simulink model "LKAS_AutoSave_20220310_1755"  (R2018b)
settings: Solver=FixedStepDiscrete  StartTime=0.0  StopTime=10.0  FixedStep=0.01  RelTol=1e-3
InitFcn:
  | tmpVer = ver('MATLAB');
  | tmpVer = str2num(tmpVer.Version);
  | % -------------------------------------------------------------------
  | %  MATLAB file generated by Simulink.saveVars on 21-Nov-2019 10:06:14
  | %  MATLAB version: 7.13.0.564 (R2011b)
  | % -------------------------------------------------------------------
  | 
  | 
  | SInt16 = Simulink.AliasType;
  | SInt16.Description = 'Num';
  | if (tmpVer > 7.11)
  | 	SInt16.DataScope = 'Auto';
  | end
  | SInt16.HeaderFile = 'Rte_Type.h';
  | SInt16.BaseType = 'int16';
  | 
  | SInt32 = Simulink.AliasType;
  | SInt32.Description = 'Num';
  | if (tmpVer > 7.11)
  | 	SInt32.DataScope = 'Auto';
  | end
  | SInt32.HeaderFile = 'Rte_Type.h';
  | SInt32.BaseType = 'int32';
  | 
  | SInt8 = Simulink.AliasType;
  | SInt8.Description = 'Num';
  | if (tmpVer > 7.11)
  | 	SInt8.DataScope = 'Auto';
  | end
  | SInt8.HeaderFile = 'Rte_Type.h';
  | SInt8.BaseType = 'int8';
  | 
  | T_A_m2_1024_1_u32 = Simulink.NumericType;
  | T_A_m2_1024_1_u32.Description = 'm2 (square meters  (m2))';
  | if (tmpVer > 7.11)
  | 	T_A_m2_1024_1_u32.DataScope = 'Auto';
  | end
  | T_A_m2_1024_1_u32.HeaderFile = 'Rte_Type.h';
  | T_A_m2_1024_1_u32.DataTypeMode = 'Fixed-point: slope and bias scaling';
  | T_A_m2_1024_1_u32.SignednessBool = false;
  | T_A_m2_1024_1_u32.WordLength = 32;
  | T_A_m2_1024_1_u32.FixedExponent = -10;
  | T_A_m2_1024_1_u32.SlopeAdjustmentFactor = 1;
  | T_A_m2_1024_1_u32.Bias = 0;
  | T_A_m2_1024_1_u32.DataTypeOverride = 'Inherit';
  | T_A_m2_1024_1_u32.IsAlias = true;
  | 
  | T_A_m2_65536_1_u16 = Simulink.NumericType;
  | T_A_m2_65536_1_u16.Description = 'm2 (square meters  (m2))';
  | if (tmpVer > 7.11)
  | 	T_A_m2_65536_1_u16.DataScope = 'Auto';
  | end
  | T_A_m2_65536_1_u16.HeaderFile = 'Rte_Type.h';
  | T_A_m2_65536_1_u16.DataTypeMode = 'Fixed-point: slope and bias scaling';
  | T_A_m2_65536_1_u16.SignednessBool = false;
  | T_A_m2_65536_1_u16.WordLength = 16;
  | T_A_m2_65536_1_u16.FixedExponent = -16;
  | T_A_m2_65536_1_u16.SlopeAdjustmentFactor = 1;
  | T_A_m2_65536_1_u16.Bias = 0;
  | T_A_m2_65536_1_u16.DataTypeOverride = 'Inherit';
  | ... (+4647 lines)
StopFcn:
  | clear  T_A_m2_1024_1_u32 T_A_m2_65536_1_u16 T_A_m2_Float32 T_A_mm2_10_1_u16 T_A_mm2_4_1_s16 T_A_mm2_Float32 T_Cnt_Num_10_1_u32 T_Cnt_Num_1_1_s16 T_Cnt_Num_1_1_s32 T_Cnt_Num_1_1_s8 T_Cnt_Num_1_1_u16 T_Cnt_Num_1_1_u32 T_Cnt_Num_1_1_u8 T_E_J_1_1_s32 T_E_J_Float32 T_E_kJ_128_1_s32 T_E_kJ_Float32 T_E_kwh_10_1_u16 T_E_kwh_Float32 T_Epl_kwhpkm_100_1_u16 T_Epl_kwhpkm_Float32 T_F_N_1_1_s16 T_F_N_Float32 T_I_A_1000_1_u16 T_I_A_1048576_1_s32 T_I_A_2048_1_s16 T_I_A_32_1_s16 T_I_A_Float32 T_I_mA_1_1_s16 T_I_mA_32768_128_s16 T_I_mA_Float32 T_J_kgpm2_128_1_u16 T_J_kgpm2_Float32 T_K_NA_1000_1_s16 T_K_NA_100_1_s16 T_K_NA_100_1_u16 T_K_NA_1024_1_s16 T_K_NA_1024_1_u16 T_K_NA_128_1_s16 T_K_NA_128_1_u16 T_K_NA_128_1_u8 T_K_NA_16777216_1_u32 T_K_NA_16_1_s16 T_K_NA_16_1_u16 T_K_NA_16_1_u8 T_K_NA_1_16_u16 T_K_NA_1_1_s16 T_K_NA_1_1_u16 T_K_NA_1_1_u8 T_K_NA_32768_1_s16 T_K_NA_32768_1_u16 T_K_NA_32_1_s8 T_K_NA_4096_1_u16 T_K_NA_4194304_1_s32 T_K_NA_4194304_1_u16 T_K_NA_65536_1_s32 T_K_NA_65536_1_u16 T_K_NA_8192_1_s16 T_K_NA_8_1_s16 T_K_NA_Float32 T_M_Nm_16_1_s16 T_M_Nm_1_1_s16 T_M_Nm_32768_1_s16 T_M_Nm_32_1_s16 T_M_Nm_4_1_s16 T_M_Nm_512_1_s16 T_M_Nm_Float32 T_P_W_1_4_s16 T_P_W_1_8_s16 T_P_W_Float32 T_P_kW_128_1_s16 T_P_kW_1_8_s16 T_P_kW_8_1_s32 T_P_kW_Float32 T_Pct_pct_1024_1_s32 T_Pct_pct_1024_1_u32 T_Pct_pct_10_1_s16 T_Pct_pct_10_1_u32 T_Pct_pct_128_100_s8 T_Pct_pct_1_1_s16 T_Pct_pct_1_4_u8 T_Pct_pct_255_100_u16 T_Pct_pct_255_100_u8 T_Pct_pct_256_1_s16 T_Pct_pct_256_1_u16 T_Pct_pct_65535_100_u16 T_Pct_pct_Float32 T_R_ohm_1024_1_s16 T_R_ohm_32_1_s16 T_R_ohm_Float32 T_TK_K_16_1_s16 T_TK_K_Float32 T_T_degC_10_400_1_u16 T_T_degC_16_1_s16 T_T_degC_1_40_1_u8 T_T_degC_2_80_1_u8 T_T_degC_Float32 T_U_V_1000_1_u16 T_U_V_10_1_u8 T_U_V_200_1_u8 T_U_V_32_1_s16 T_U_V_4096_1_s16 T_U_V_512_1_s16 T_U_V_65535_8_u16 T_U_V_8192_1_u16 T_U_V_Float32 T_U_mV_1_1_s16 T_U_mV_256_20_u16 T_U_mV_Float32 T_V_l_256_1_s16 T_V_l_4096_1_s16 T_V_l_64_1_s16 T_V_l_65535_100_u16 T_V_l_Float32 T_V_ml_128_1_s16 T_V_ml_1_1_s16 T_V_ml_32768_1_s16 T_V_ml_Float32 T_V_ul_32_1_u16 T_V_ul_Float32 T_Vpl_clpkm_512_1_u16 T_Vpl_clpkm_Float32 T_a_kphps_16_1_s16 T_a_kphps_Float32 T_a_mps2_128_1_s16 T_a_mps2_Float32 T_c_MJpkg_256_1_s16 T_c_MJpkg_Float32 T_c_kJpgpK_1024_1_s16 T_c_kJpgpK_Float32 T_c_kJpkgpK_128_1_u16 T_c_kJpkgpK_Float32 T_chrg_Ah_1_1_s16 T_chrg_Ah_1_1_u16 T_chrg_Ah_1_1_u8 T_chrg_Ah_256_1_u16 T_chrg_Ah_4194304_1_s32 T_chrg_Ah_512_1_u16 T_chrg_Ah_8_1_u16 T_chrg_Ah_Float32 T_cmp_NA_100_1_s16 T_cmp_NA_128_1_s16 T_cmp_NA_16_1_s16 T_cmp_NA_32768_1_u16 T_cmp_NA_Float32 T_d2n_rpmps2_4_1_s16 T_d2n_rpmps2_Float32 T_dPct_pctps_16_1_s16 T_dPct_pctps_256_1_s16 T_dPct_pctps_Float32 T_dT_degCps_128_1_s16 T_dT_degCps_Float32 T_dV_lph_1_1_s16 T_dV_lph_Float32 T_dV_lpm_128_1_s16 T_dV_lpm_32_1_s16 T_dV_lpm_Float32 T_dV_lps_1024_1_u16 T_dV_lps_4_1_u16 T_dV_lps_Float32 T_dV_mlps_1024_1_s16 T_dV_mlps_Float32 T_d_BitField16 T_dm_gps_128_1_s16 T_dm_gps_128_1_u16 T_dm_gps_256_1_u16 T_dm_gps_Float32 T_dm_mgps_1_1_s16 T_dm_mgps_Float32 T_dn_rpmps_1_1_s16 T_dn_rpmps_2_1_s16 T_dn_rpmps_Float32 T_dp_Paps_1_1_s16 T_dp_Paps_Float32 T_dp_kPaps_1_1_s16 T_dp_kPaps_8_1_s16 T_dp_kPaps_Float32 T_dphi_degps_128_1_s16 T_dphi_degps_8_1_s16 T_dphi_degps_Float32 T_dr_ps_256_1_s16 T_dr_ps_Float32 T_drho_mgplps_1_2_s16 T_drho_mgplps_Float32 T_e_NA_1_1_u8 T_f_Hz_1_1_u16 T_f_Hz_1_1_u32 T_f_Hz_64_1_u16 T_f_Hz_8_1_s16 T_f_Hz_Float32 T_g_BitField32 T_l_km_16_1_s16 T_l_km_1_1_u16 T_l_km_1_1_u32 T_l_km_Float32 T_l_m_1024_1_s16 T_l_m_16_1_s16 T_l_m_1_1_u32 T_l_m_Float32 T_l_mm_16_1_s16 T_l_mm_1_1_u16 T_l_mm_4096_1_s16 T_l_mm_4_1_u8 T_l_mm_64_1_s16 T_l_mm_Float32 T_m_g_1_1_s16 T_m_g_2048_1_s16 T_m_g_32_1_u16 T_m_g_Float32 T_m_kg_1024_1_s16 T_m_kg_1_1_s16 T_m_kg_1_1_u32 T_m_kg_Float32 T_m_mg_128_1_s16 T_m_mg_32_1_s16 T_m_mg_Float32 T_n_rpm_1_1_s16 T_n_rpm_1_25_u8 T_n_rpm_256_50_u16 T_n_rpm_2_25_u8 T_n_rpm_4_1_u16 T_n_rpm_Float32 T_p_MPa_64_1_s16 T_p_MPa_Float32 T_p_Pa_1_1_s16 T_p_Pa_Float32 T_p_kPa_1_10_u16 T_p_kPa_1_1_s16 T_p_kPa_1_1_u8 T_p_kPa_256_1_u16 T_p_kPa_32_1_u16 T_p_kPa_64_1_s16 T_p_kPa_Float32 T_phi_deg_100_1_s16 T_phi_deg_1024_1_s16 T_phi_deg_128_1_s16 T_phi_deg_1_1_u8 T_phi_deg_256_1_s16 T_phi_deg_2_1_s8 T_phi_deg_32_1_s16 T_phi_deg_512_6_s32 T_phi_deg_Float32 T_phi_rad_2048_1_s16 T_phi_rad_Float32 T_r_NA_1024_1_s16 T_r_NA_1024_1_u16 T_r_NA_16384_1_s16 T_r_NA_16_1_s16 T_r_NA_256_1_s8 T_r_NA_256_1_u16 T_r_NA_32768_1_u16 T_r_NA_32_1_u16 T_r_NA_4096_1_s16 T_r_NA_65535_2_u16 T_r_NA_8192_1_u16 T_r_NA_Float32 T_rho_gpl_8192_1_s16 T_rho_gpl_Float32 T_rho_kgpm3_16_1_s16 T_rho_kgpm3_Float32 T_rho_mgpl_1_1_s16 T_rho_mgpl_64_1_s16 T_rho_mgpl_Float32 T_t_hour_1_1_s16 T_t_hour_Float32 T_t_m_1_1_u16 T_t_m_Float32 T_t_ms_1_1_s16 T_t_ms_1_1_u16 T_t_ms_1_1_u32 T_t_ms_4096_1_s16 T_t_ms_64_1_s16 T_t_ms_Float32 T_t_s_1000_1_s16 T_t_s_100_1_s16 T_t_s_10_1_s16 T_t_s_10_1_u16 T_t_s_1_1_s16 T_t_s_1_1_u16 T_t_s_1_1_u32 T_t_s_Float32 T_t_us_10_1_u32 T_t_us_1_1_s16 T_t_us_1_1_u32 T_t_us_1_4_u16 T_t_us_Float32 T_v_kph_1_1_u8 T_v_kph_64_1_s16 T_v_kph_64_1_u16 T_v_kph_Float32 T_v_mps_256_1_s16 T_v_mps_Float32 T_w_radps_32_1_s16 T_w_radps_Float32 T_y_BitField8 T_y_BitFieldDiagProgress T_y_BitFieldDiagStatus T_y_NA_1_1_u8 SInt16 SInt32 SInt8 T_BOOLEAN UInt16 UInt32 UInt8 s16 s32 s8 u16 u32 u8
model workspace (MAT data in the model file):
  MCOS : class17 (value not decoded)
  MCOS : class17 (value not decoded)
  MCOS : class17 (value not decoded)
  MCOS : class17 (value not decoded)
  MCOS : class17 (value not decoded)
  MCOS : class17 (value not decoded)
  MCOS : class17 (value not decoded)
  MCOS : class17 (value not decoded)
  MCOS : class17 (value not decoded)
  MCOS : class17 (value not decoded)
  MCOS : class17 (value not decoded)
  MCOS : class17 (value not decoded)
  MCOS : class17 (value not decoded)
  MCOS : class17 (value not decoded)
  MCOS : class17 (value not decoded)
  MCOS : class17 (value not decoded)
  MCOS : class17 (value not decoded)
  MCOS : class17 (value not decoded)
  MCOS : class17 (value not decoded)
  MCOS : class17 (value not decoded)
  MCOS : class17 (value not decoded)
  MCOS : class17 (value not decoded)
  MCOS : class17 (value not decoded)
  MCOS : class17 (value not decoded)
  MCOS : class17 (value not decoded)
  MCOS : class17 (value not decoded)
  MCOS : class17 (value not decoded)
  MCOS : class17 (value not decoded)
  MCOS : class17 (value not decoded)
  MCOS : class17 (value not decoded)
  MCOS : class17 (value not decoded)
  MCOS : class17 (value not decoded)
  MCOS : class17 (value not decoded)
  MCOS : class17 (value not decoded)
  MCOS : class17 (value not decoded)
  MCOS : class17 (value not decoded)
  MCOS : class17 (value not decoded)
  MCOS : class17 (value not decoded)
  MCOS : class17 (value not decoded)
  MCOS : class17 (value not decoded)
  MCOS : class17 (value not decoded)
  MCOS : class17 (value not decoded)
  MCOS : class17 (value not decoded)
  MCOS : class17 (value not decoded)
  MCOS : class17 (value not decoded)
  MCOS : class17 (value not decoded)
  MCOS : class17 (value not decoded)
  MCOS : class17 (value not decoded)
  MCOS : class17 (value not decoded)
  MCOS : class17 (value not decoded)
  MCOS : class17 (value not decoded)
  MCOS : class17 (value not decoded)
  MCOS : class17 (value not decoded)
  MCOS : class17 (value not decoded)
  MCOS : class17 (value not decoded)
  MCOS : class17 (value not decoded)
  MCOS : class17 (value not decoded)
  MCOS : class17 (value not decoded)
  MCOS : class17 (value not decoded)
  MCOS : class17 (value not decoded)
  MCOS : class17 (value not decoded)
  MCOS : class17 (value not decoded)
  MCOS : class17 (value not decoded)
  MCOS : class17 (value not decoded)
  MCOS : class17 (value not decoded)
  MCOS : class17 (value not decoded)
  MCOS : class17 (value not decoded)
  MCOS : class17 (value not decoded)
  MCOS : class17 (value not decoded)
  MCOS : class17 (value not decoded)
  MCOS : class17 (value not decoded)
  MCOS : class17 (value not decoded)
  MCOS : class17 (value not decoded)
  MCOS : class17 (value not decoded)
  MCOS : class17 (value not decoded)
  MCOS : class17 (value not decoded)
  MCOS : class17 (value not decoded)
  MCOS : class17 (value not decoded)
  MCOS : class17 (value not decoded)
  MCOS : class17 (value not decoded)
  MCOS : class17 (value not decoded)
  MCOS : class17 (value not decoded)
  MCOS : class17 (value not decoded)
  MCOS : class17 (value not decoded)
  MCOS : class17 (value not decoded)
  MCOS : class17 (value not decoded)
  MCOS : class17 (value not decoded)
  MCOS : class17 (value not decoded)
  MCOS : class17 (value not decoded)
  MCOS : class17 (value not decoded)
  MCOS : class17 (value not decoded)
  MCOS : class17 (value not decoded)
  MCOS : class17 (value not decoded)
  MCOS : class17 (value not decoded)
  MCOS : class17 (value not decoded)
  MCOS : class17 (value not decoded)
  MCOS : class17 (value not decoded)
  MCOS : class17 (value not decoded)
  MCOS : class17 (value not decoded)
  MCOS : class17 (value not decoded)
  MCOS : class17 (value not decoded)
  MCOS : class17 (value not decoded)
undefined symbols (not defined in the file): LKA_CarWidth, LKA_SampleTime, LKA_StrRatio_C, LKA_Veh2CamL_C, LKA_Veh2CamW_C, LKA_WhlBaseL_C, LL_CompHdAg_C, LL_CompSWA_C, LL_CrvtPrvwT_C, LL_DesDvt_C, LL_DvtComp_C, LL_DvtPrvwT_C, LL_DvtSpdDet_vDvtSpdMin_C, LL_HandsOff_ExitTime, LL_HandsOff_TextTime, LL_HandsOff_WarnTime, LL_HdAgExT_C, LL_HdAgPrvwT_C, LL_LAccMax_C, LL_LAccRMax_C, LL_LDW_EarliestWarnLine_C, LL_LDW_LatestWarnLine_C, LL_LDWS_SUPPRESS_HEADING, LL_LFClb_TFC_FfCtlRatio_C, LL_LFClb_TFC_KdBalance_C, LL_LFClb_TFC_KdMaxSWA_C, LL_LFClb_TFC_KdV1_C, LL_LFClb_TFC_KdV2_C, LL_LFClb_TFC_KdVehSpdLwr_C, LL_LFClb_TFC_KdVehSpdUpr_C, LL_LFClb_TFC_Ki_C, LL_LFClb_TFC_KiMaxSWA_C, LL_LFClb_TFC_Kp_C, LL_LFClb_TFC_KpKlat_C, LL_LFClb_TFC_KpV1_C, LL_LFClb_TFC_KpV2_C, LL_LFClb_TFC_KpVehSpdLwr_C, LL_LFClb_TFC_KpVehSpdUpr_C, LL_LFClb_TFC_PrvwT_C, LL_LKA_EarliestWarnLine_C, LL_LKA_LatestWarnLine_C, LL_LKAExPrcs_ExitC0Dvt, LL_LKAExPrcs_ExitC0Swt, LL_LKAExPrcs_tiExitTime1, LL_LKAExPrcs_tiExitTime2, LL_LKAExPrcs_tiExitTime3, LL_LKAS_OUT_OF_CONTROL_LAT_VEL, LL_LKAS_OUT_OF_CONTROL_TTLC, LL_LKASWASyn_M0, LL_LKASWASyn_M1, LL_LKASWASyn_M2, LL_LKASWASyn_M3K, LL_LKASWASyn_SWAaddMax, LL_LKASWASyn_T2, LL_LKASWASyn_tiTrqSwaRtTime, LL_LKASWASyn_tiTrqSwaTime, LL_LKASWASyn_TrqMax, LL_LKASWASyn_TrqSwaAddSwt, LL_LKASWASyn_TrqSwaRateDiff, LL_LSpdCompT_C ... (+43)
libraries: simulink x138, canmsglib x8, dspstat3 x3, simulink_extras x1
(part 6 of 20)

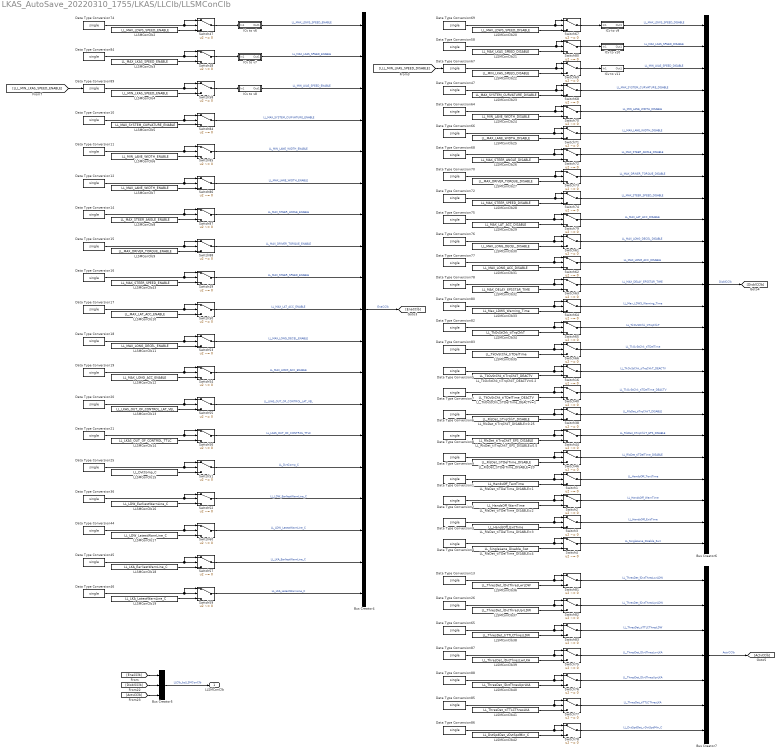
== system LKAS_AutoSave_20220310_1755/LKAS/LLClb/LLSMConClb ==
  Bus Creator4 : BusCreator  Inputs=19
  Bus Creator5 : BusCreator  Inputs=3
  Bus Creator6 : BusCreator  Inputs=25
  Bus Creator7 : BusCreator  Inputs=7
  Data Type Conversion{1..21,25..26,36,44..47,58,64..70,72,74..78,80,82..89} (51 alike) : DataTypeConversion  OutDataTypeStr=single
  ICv to v10 : Subsystem
  ICv to v11 : Subsystem
  ICv to v6 : Subsystem  Description=|
      | 仪表车速转换
      | 仪表车速 = 实际车速 * 1.02 + 2.5
      settings: AttributesFormatString=%<Description>
  ICv to v7 : Subsystem
  ICv to v8 : Subsystem
  ICv to v9 : Subsystem
  LLSMConClb10 : Constant  Description=侧向加速度使能上限  Value=LL_MAX_LAT_ACC_ENABLE  OutDataTypeStr=single
      settings: AttributesFormatString=|
      | %<Value>  = 3
      | %<Description>
  LLSMConClb11 : Constant  Description=纵向减速度使能上限  Value=LL_MAX_LONG_DECEL_ENABLE  OutDataTypeStr=single
      settings: AttributesFormatString=|
      | %<Value>  = 2
      | %<Description>
  LLSMConClb12 : Constant  Description=纵向加速度使能上限  Value=LL_MAX_LONG_ACC_ENABLE  OutDataTypeStr=single
      settings: AttributesFormatString=|
      | %<Value>  = 3
      | %<Description>
  LLSMConClb13 : Constant  Description=LKA功能的侧向偏出速度阈值  Value=LL_LKAS_OUT_OF_CONTROL_LAT_VEL  OutDataTypeStr=single
      settings: AttributesFormatString=|
      | %<Value>  = 1.5
      | %<Description>
  LLSMConClb14 : Constant  Description=LKA功能的超过最迟干预线持续时间阈值  Value=LL_LKAS_OUT_OF_CONTROL_TTLC  OutDataTypeStr=single
      settings: AttributesFormatString=|
      | %<Value>  = 0.3
      | %<Description>
  LLSMConClb15 : Constant  Description=偏移量补偿  Value=LL_DvtComp_C  OutDataTypeStr=single
      settings: AttributesFormatString=|
      | %<Value>  = 0
      | %<Description>
  LLSMConClb16 : Constant  Description=LDW功能的最早预警线  Value=LL_LDW_EarliestWarnLine_C  OutDataTypeStr=single
      settings: AttributesFormatString=|
      | %<Value>  = 0.3
      | %<Description>
  LLSMConClb17 : Constant  Description=LDW功能的最迟预警线  Value=LL_LDW_LatestWarnLine_C  OutDataTypeStr=single
      settings: AttributesFormatString=|
      | %<Value>  = -0.4
      | %<Description>
  LLSMConClb18 : Constant  Description=LKA功能的最早预警线  Value=LL_LKA_EarliestWarnLine_C  OutDataTypeStr=single
      settings: AttributesFormatString=|
      | %<Value>  = 0.3
      | %<Description>
  LLSMConClb19 : Constant  Description=LKA功能的最迟预警线  Value=LL_LKA_LatestWarnLine_C  OutDataTypeStr=single
      settings: AttributesFormatString=|
      | %<Value>  = -0.5
      | %<Description>
  LLSMConClb2 : Constant  Description=LDW功能的车速使能上限  Value=LL_MAX_LDWS_SPEED_ENABLE  OutDataTypeStr=single
      settings: AttributesFormatString=|
      | %<Value>  = 140
      | %<Description>
  LLSMConClb20 : Constant  Description=LDW功能的车速失效上限  Value=LL_MAX_LDWS_SPEED_DISABLE  OutDataTypeStr=single
      settings: AttributesFormatString=|
      | %<Value>  = 150
      | %<Description>
  LLSMConClb21 : Constant  Description=LKA功能的车速失效上限  Value=LL_MAX_LKAS_SPEED_DISABLE  OutDataTypeStr=single
      settings: AttributesFormatString=|
      | %<Value>  = 150
      | %<Description>
  LLSMConClb22 : Constant  Description=LKA功能的车速失效下限  Value=LL_MIN_LKAS_SPEED_DISABLE  OutDataTypeStr=single
      settings: AttributesFormatString=|
      | %<Value>  = 55
      | %<Description>
  LLSMConClb23 : Constant  Description=曲率失效上限  Value=LL_MAX_SYSTEM_CURVATURE_DISABLE  OutDataTypeStr=single
      settings: AttributesFormatString=|
      | %<Value>  = 0.0055
      | %<Description>
  LLSMConClb24 : Constant  Description=车道线宽度失效下限  Value=LL_MIN_LANE_WIDTH_DISABLE  OutDataTypeStr=single
      settings: AttributesFormatString=|
      | %<Value>  = 2.4
      | %<Description>
  LLSMConClb25 : Constant  Description=车道线宽度失效上限  Value=LL_MAX_LANE_WIDTH_DISABLE  OutDataTypeStr=single
      settings: AttributesFormatString=|
      | %<Value>  = 5.5
      | %<Description>
  LLSMConClb26 : Constant  Description=方向盘转角退出上限  Value=LL_MAX_STEER_ANGLE_DISABLE  OutDataTypeStr=single
      settings: AttributesFormatString=|
      | %<Value>  = 70
      | %<Description>
  LLSMConClb27 : Constant  Description=驾驶员转矩失效上限  Value=LL_MAX_DRIVER_TORQUE_DISABLE  OutDataTypeStr=single
      settings: AttributesFormatString=|
      | %<Value>  = 2.25
      | %<Description>
  LLSMConClb28 : Constant  Description=方向盘转速失效上限  Value=LL_MAX_STEER_SPEED_DISABLE  OutDataTypeStr=single
      settings: AttributesFormatString=|
      | %<Value>  = 5000
      | %<Description>
  LLSMConClb29 : Constant  Description=侧向加速度失效上限  Value=LL_MAX_LAT_ACC_DISABLE  OutDataTypeStr=single
      settings: AttributesFormatString=|
      | %<Value>  = 3.5
      | %<Description>
  LLSMConClb3 : Constant  Description=LKA功能的车速使能上限  Value=LL_MAX_LKAS_SPEED_ENABLE  OutDataTypeStr=single
      settings: AttributesFormatString=|
      | %<Value>  = 140
      | %<Description>
  LLSMConClb30 : Constant  Description=纵向减速度失效上限  Value=LL_MAX_LONG_DECEL_DISABLE  OutDataTypeStr=single
      settings: AttributesFormatString=|
      | %<Value>  = 2.5
      | %<Description>
  LLSMConClb31 : Constant  Description=纵向加速度失效上限  Value=LL_MAX_LONG_ACC_DISABLE  OutDataTypeStr=single
      settings: AttributesFormatString=|
      | %<Value>  = 3.5
      | %<Description>
  LLSMConClb32 : Constant  Description=LKA功能的EPS延迟进入等待的时间上限  Value=LL_MAX_DELAY_EPSSTAR_TIME  OutDataTypeStr=single
      settings: AttributesFormatString=|
      | %<Value>  = 0.5
      | %<Description>
  LLSMConClb33 : Constant  Description=LDW功能的连续报警时间上限  Value=LL_Max_LDWS_Warning_Time  OutDataTypeStr=single
      settings: AttributesFormatString=|
      | %<Value>  = 5
      | %<Description>
  LLSMConClb34 : Constant  Description=驾驶员接管时间阈值  Value=LL_TkOvStChk_tiTrqChkT  OutDataTypeStr=single
      settings: AttributesFormatString=|
      | %<Value>  = 0.1
      | %<Description>
  LLSMConClb35 : Constant  Description=距离上次驾驶员接管时间间隔  Value=LL_TkOvStChk_tiTDelTime  OutDataTypeStr=single
      settings: AttributesFormatString=|
      | %<Value>  = 2
      | %<Description>
  LLSMConClb36 : Constant  Description=LDW功能的偏移量激活下限  Value=LL_ThresDet_lDvtThresLwrLDW  OutDataTypeStr=single
      settings: AttributesFormatString=|
      | %<Value>  = 0.15
      | %<Description>
  LLSMConClb37 : Constant  Description=LDW功能的偏移量激活上限  Value=LL_ThresDet_lDvtThresUprLDW  OutDataTypeStr=single
      settings: AttributesFormatString=|
      | %<Value>  = 0.3
      | %<Description>
  LLSMConClb38 : Constant  Description=LDW功能的跨道时间激活阈值  Value=LL_ThresDet_tiTTLCThresLDW  OutDataTypeStr=single
      settings: AttributesFormatString=|
      | %<Value>  = 0.75
      | %<Description>
  LLSMConClb39 : Constant  Description=LKA功能的偏移量激活下限  Value=LL_ThresDet_lDvtThresLwrLKA  OutDataTypeStr=single
      settings: AttributesFormatString=|
      | %<Value>  = 0.3
      | %<Description>
  LLSMConClb4 : Constant  Description=LKA功能的车速使能下限  Value=LL_MIN_LKAS_SPEED_ENABLE  OutDataTypeStr=single
      settings: AttributesFormatString=|
      | %<Value>  = 60
      | %<Description>
  LLSMConClb40 : Constant  Description=LKA功能的偏移量激活上限  Value=LL_ThresDet_lDvtThresUprLKA  OutDataTypeStr=single
      settings: AttributesFormatString=|
      | %<Value>  = 0.6
      | %<Description>
  LLSMConClb41 : Constant  Description=LKA功能的跨道时间激活阈值  Value=LL_ThresDet_tiTTLCThresLKA  OutDataTypeStr=single
      settings: AttributesFormatString=|
      | %<Value>  = 1.5
      | %<Description>
  LLSMConClb42 : Constant  Description=偏出侧向速度最小值  Value=LL_DvtSpdDet_vDvtSpdMin_C  OutDataTypeStr=single
      settings: AttributesFormatString=|
      | %<Value>  = 0
      | %<Description>
  LLSMConClb43 : Constant  Description=方向盘转速使能上限  Value=LL_MAX_STEER_SPEED_ENABLE  OutDataTypeStr=single
      settings: AttributesFormatString=|
      | %<Value>  = 5000
      | %<Description>
  LLSMConClb5 : Constant  Description=曲率使能上限  Value=LL_MAX_SYSTEM_CURVATURE_ENABLE  OutDataTypeStr=single
      settings: AttributesFormatString=|
      | %<Value>  = 0.0045
      | %<Description>
  LLSMConClb6 : Constant  Description=车道线宽度使能下限  Value=LL_MIN_LANE_WIDTH_ENABLE  OutDataTypeStr=single
      settings: AttributesFormatString=|
      | %<Value>  = 2.5
      | %<Description>
  LLSMConClb7 : Constant  Description=车道线宽度使能上限  Value=LL_MAX_LANE_WIDTH_ENABLE  OutDataTypeStr=single
      settings: AttributesFormatString=|
      | %<Value>  = 5.4
      | %<Description>
  LLSMConClb8 : Constant  Description=方向盘转角使能上限  Value=LL_MAX_STEER_ANGLE_ENABLE  OutDataTypeStr=single
      settings: AttributesFormatString=|
      | %<Value>  = 60
      | %<Description>
  LLSMConClb9 : Constant  Description=驾驶员扭矩使能上限  Value=LL_MAX_DRIVER_TORQUE_ENABLE  OutDataTypeStr=single
      settings: AttributesFormatString=|
      | %<Value>  = 3
      | %<Description>
  LL_RlsDet_tiTDelTime_DISABLE=1 : Constant  Description=驾驶员脱手开始到功能发出动画提醒的时间  Value=LL_HandsOff_TextTime  OutDataTypeStr=single
      settings: AttributesFormatString=|
      | %<Value>  = 10
      | %<Description>
  LL_RlsDet_tiTDelTime_DISABLE=2 : Constant  Description=驾驶员脱手开始到发出声音报警的时间  Value=LL_HandsOff_WarnTime  OutDataTypeStr=single
      settings: AttributesFormatString=|
      | %<Value>  = 15
      | %<Description>
  LL_RlsDet_tiTDelTime_DISABLE=20 : Constant  Description=反使能距离上次驾驶员脱手时间间隔  Value=LL_RlsDet_tiTDelTime_DISABLE  OutDataTypeStr=single
      settings: AttributesFormatString=|
      | %<Value>  = 20
      | %<Description>
  LL_RlsDet_tiTDelTime_DISABLE=3 : Constant  Description=驾驶员脱手开始到功能退出的时间  Value=LL_HandsOff_ExitTime  OutDataTypeStr=single
      settings: AttributesFormatString=|
      | %<Value>  = 20
      | %<Description>
  LL_RlsDet_tiTDelTime_DISABLE=4 : Constant  Description=驾驶员脱手开始到功能退出的时间  Value=LL_SingleLane_Disable_Swt  OutDataTypeStr=boolean
      settings: AttributesFormatString=|
      | %<Value>  = 0
      | %<Description>
  LL_RlsDet_tiTrqChkT_DISABLE=0.25 : Constant  Description=反使能驾驶员脱手时间阈值  Value=LL_RlsDet_tiTrqChkT_DISABLE  OutDataTypeStr=single
      settings: AttributesFormatString=|
      | %<Value>  = 0.25
      | %<Description>
  LL_RlsDet_tiTrqChkT_EPS_DISABLE=0.5 : Constant  Description=反使能驾驶员脱手时间阈值（EPS激活）  Value=LL_RlsDet_tiTrqChkT_EPS_DISABLE  OutDataTypeStr=single
      settings: AttributesFormatString=|
      | %<Value>  = 0.5
      | %<Description>
  LL_TkOvStChk_tiTDelTime_DEACTV=1 : Constant  Description=取消激活距离上次驾驶员接管时间间隔  Value=LL_TkOvStChk_tiTDelTime_DEACTV  OutDataTypeStr=single
      settings: AttributesFormatString=|
      | %<Value>  = 1
      | %<Description>
  LL_TkOvStChk_tiTrqChkT_DEACTV=0.2 : Constant  Description=取消激活驾驶员接管时间阈值  Value=LL_TkOvStChk_tiTrqChkT_DEACTV  OutDataTypeStr=single
      settings: AttributesFormatString=|
      | %<Value>  = 0.2
      | %<Description>
  Switch{1..3,16,38,40,44,46..88} (50 alike) : Switch  Criteria=u2 ~= 0  OutDataTypeStr=single
  Switch4 : Switch  Criteria=u2 ~= 0  OutDataTypeStr=boolean
  LLSMConClb : Outport
  wires:
  Bus Creator5/1 -> LLSMConClb/1  "LLClb_bsLLSMConClb"
  [ActvCClb] -> Bus Creator5/3
  [DisblCClb] -> Bus Creator5/2
  [EnaCClb] -> Bus Creator5/1
  ICv to v6/1(Out1) -> Bus Creator4/1  "LL_MAX_LDWS_SPEED_ENABLE"
  LLSMConClb3/1 -> Switch48/3
  LLSMConClb10/1 -> Switch50/3
  LLSMConClb41/1 -> Switch77/3
  Data Type Conversion66/1 -> Switch71/1, Switch71/2
  LLSMConClb39/1 -> Switch75/3
  LLSMConClb11/1 -> Switch53/3
  LLSMConClb12/1 -> Switch54/3
  Switch55/1 -> Bus Creator4/13  "LL_LKAS_OUT_OF_CONTROL_LAT_VEL"
  Switch82/1 -> Bus Creator7/2  "LL_ThresDet_lDvtThresUprLDW"
  Data Type Conversion46/1 -> Switch59/1, Switch59/2
  Bus Creator7/1 -> [ActvCClb]  "ActvCClb"
  [LLL_MIN_LKAS_SPEED_DISABLE] -> Data Type Conversion67/1
  Data Type Conversion65/1 -> Switch83/2, Switch83/1
  ICv to v9/1(Out1) -> Bus Creator6/1  "LL_MAX_LDWS_SPEED_DISABLE"
  Switch69/1 -> ICv to v11/1(In1)
  LLSMConClb38/1 -> Switch83/3
  Data Type Conversion17/1 -> Switch50/1, Switch50/2
  Data Type Conversion78/1 -> Switch63/1, Switch63/2
  Data Type Conversion14/1 -> Switch87/1, Switch87/2
  ICv to v7/1(Out1) -> Bus Creator4/2  "LL_MAX_LKAS_SPEED_ENABLE"
  LLSMConClb35/1 -> Switch66/3
  Data Type Conversion64/1 -> Switch70/1, Switch70/2
  LLSMConClb14/1 -> Switch56/3
  Data Type Conversion69/1 -> Switch67/1, Switch67/2
  LLSMConClb5/1 -> Switch84/3
  LLSMConClb37/1 -> Switch82/3
  Data Type Conversion70/1 -> Switch73/1, Switch73/2
  Switch85/1 -> Bus Creator4/5  "LL_MIN_LANE_WIDTH_ENABLE"
  LLSMConClb23/1 -> Switch68/3
  Switch59/1 -> Bus Creator4/19  "LL_LKA_LatestWarnLine_C"
  LLSMConClb25/1 -> Switch71/3
  LLSMConClb43/1 -> Switch49/3
  Switch49/1 -> Bus Creator4/9  "LL_MAX_STEER_SPEED_ENABLE"
  LLSMConClb40/1 -> Switch76/3
  Switch50/1 -> Bus Creator4/10  "LL_MAX_LAT_ACC_ENABLE"
  Data Type Conversion68/1 -> Switch72/1, Switch72/2
  LLSMConClb33/1 -> Switch64/3
  Switch81/1 -> Bus Creator7/1  "LL_ThresDet_lDvtThresLwrLDW"
  Data Type Conversion18/1 -> Switch53/1, Switch53/2
  Switch84/1 -> Bus Creator4/4  "LL_MAX_SYSTEM_CURVATURE_ENABLE"
  Data Type Conversion76/1 -> Switch61/2, Switch61/1
  Switch53/1 -> Bus Creator4/11  "LL_MAX_LONG_DECEL_ENABLE"
  Data Type Conversion11/1 -> Switch85/1, Switch85/2
  LLSMConClb27/1 -> Switch73/3
  Data Type Conversion84/1 -> Switch48/1, Switch48/2
  Switch70/1 -> Bus Creator6/5  "LL_MIN_LANE_WIDTH_DISABLE"
  LLSMConClb34/1 -> Switch65/3
  Data Type Conversion16/1 -> Switch49/1, Switch49/2
  Switch64/1 -> Bus Creator6/14  "LL_Max_LDWS_Warning_Time"
  Data Type Conversion88/1 -> Switch76/1, Switch76/2
  Data Type Conversion13/1 -> Switch81/1, Switch81/2
  Switch52/1 -> Bus Creator4/16  "LL_LDW_EarliestWarnLine_C"
  Switch79/1 -> Bus Creator6/10  "LL_MAX_LAT_ACC_DISABLE"
  Data Type Conversion72/1 -> Switch74/1, Switch74/2
  LLSMConClb18/1 -> Switch57/3
  Data Type Conversion82/1 -> Switch65/1, Switch65/2
  Data Type Conversion58/1 -> Switch80/1, Switch80/2
  Data Type Conversion19/1 -> Switch54/1, Switch54/2
  Switch51/1 -> Bus Creator4/15  "LL_DvtComp_C"
  Switch76/1 -> Bus Creator7/5  "LL_ThresDet_lDvtThresUprLKA"
  LLSMConClb7/1 -> Switch86/3
  Switch48/1 -> ICv to v7/1(In1)
  Data Type Conversion36/1 -> Switch52/1, Switch52/2
  Switch63/1 -> Bus Creator6/13  "LL_MAX_DELAY_EPSSTAR_TIME"
  LLSMConClb29/1 -> Switch79/3
  LLSMConClb21/1 -> Switch80/3
  Data Type Conversion44/1 -> Switch60/1, Switch60/2
  Switch75/1 -> Bus Creator7/4  "LL_ThresDet_lDvtThresLwrLKA"
  Bus Creator6/1 -> [DisblCClb]  "DisblCClb"
  ICv to v11/1(Out1) -> Bus Creator6/3  "LL_MIN_LKAS_SPEED_DISABLE"
  Switch80/1 -> ICv to v10/1(In1)
  LLSMConClb30/1 -> Switch61/3
  LLSMConClb24/1 -> Switch70/3
  Switch74/1 -> Bus Creator6/9  "LL_MAX_STEER_SPEED_DISABLE"
  ICv to v8/1(Out1) -> Bus Creator4/3  "LL_MIN_LKAS_SPEED_ENABLE"
  Switch77/1 -> Bus Creator7/6  "LL_ThresDet_tiTTLCThresLKA"
  LLSMConClb8/1 -> Switch87/3
  LLSMConClb16/1 -> Switch52/3
  LLSMConClb4/1 -> Switch58/3
  ICv to v10/1(Out1) -> Bus Creator6/2  "LL_MAX_LKAS_SPEED_DISABLE"
  Switch83/1 -> Bus Creator7/3  "LL_ThresDet_tiTTLCThresLDW"
  LLSMConClb26/1 -> Switch72/3
  Switch78/1 -> Bus Creator7/7  "LL_DvtSpdDet_vDvtSpdMin_C"
  LLSMConClb19/1 -> Switch59/3
  Data Type Conversion87/1 -> Switch75/2, Switch75/1
  Data Type Conversion10/1 -> Switch84/1, Switch84/2
  Switch73/1 -> Bus Creator6/8  "LL_MAX_DRIVER_TORQUE_DISABLE"
  LLSMConClb9/1 -> Switch88/3
  Switch61/1 -> Bus Creator6/11  "LL_MAX_LONG_DECEL_DISABLE"
  LLSMConClb31/1 -> Switch62/3
  Data Type Conversion77/1 -> Switch62/1, Switch62/2
  Data Type Conversion20/1 -> Switch55/1, Switch55/2
  Switch66/1 -> Bus Creator6/16  "LL_TkOvStChk_tiTDelTime"
  Switch65/1 -> Bus Creator6/15  "LL_TkOvStChk_tiTrqChkT"
  Data Type Conversion67/1 -> Switch69/2, Switch69/1
  LLSMConClb42/1 -> Switch78/3
  Data Type Conversion85/1 -> Switch77/1, Switch77/2
  Switch67/1 -> ICv to v9/1(In1)
  LLSMConClb36/1 -> Switch81/3
  LLSMConClb22/1 -> Switch69/3
  Switch54/1 -> Bus Creator4/12  "LL_MAX_LONG_ACC_ENABLE"
  LLSMConClb17/1 -> Switch60/3
  Switch47/1 -> ICv to v6/1(In1)
  LLSMConClb20/1 -> Switch67/3
  Switch87/1 -> Bus Creator4/7  "LL_MAX_STEER_ANGLE_ENABLE"
  Data Type Conversion47/1 -> Switch68/1, Switch68/2
  Data Type Conversion21/1 -> Switch56/1, Switch56/2
  Switch60/1 -> Bus Creator4/17  "LL_LDW_LatestWarnLine_C"
  LLSMConClb6/1 -> Switch85/3
  Switch62/1 -> Bus Creator6/12  "LL_MAX_LONG_ACC_DISABLE"
  Switch72/1 -> Bus Creator6/7  "LL_MAX_STEER_ANGLE_DISABLE"
  Bus Creator4/1 -> [EnaCClb]  "EnaCClb"
  Switch71/1 -> Bus Creator6/6  "LL_MAX_LANE_WIDTH_DISABLE"
  Data Type Conversion86/1 -> Switch78/2, Switch78/1
  Switch58/1 -> ICv to v8/1(In1)
  Data Type Conversion15/1 -> Switch88/1, Switch88/2
  Data Type Conversion12/1 -> Switch86/1, Switch86/2
  Data Type Conversion83/1 -> Switch66/1, Switch66/2
  Switch57/1 -> Bus Creator4/18  "LL_LKA_EarliestWarnLine_C"
  Data Type Conversion26/1 -> Switch82/2, Switch82/1
  Data Type Conversion80/1 -> Switch64/1, Switch64/2
  LLSMConClb15/1 -> Switch51/3
  LLSMConClb32/1 -> Switch63/3
  Switch68/1 -> Bus Creator6/4  "LL_MAX_SYSTEM_CURVATURE_DISABLE"
  LLSMConClb13/1 -> Switch55/3
  [LLL_MIN_LKAS_SPEED_ENABLE] -> Data Type Conversion89/1
  Data Type Conversion45/1 -> Switch57/1, Switch57/2
  LLSMConClb28/1 -> Switch74/3
  Data Type Conversion75/1 -> Switch79/2, Switch79/1
  Data Type Conversion74/1 -> Switch47/1, Switch47/2
  Switch88/1 -> Bus Creator4/8  "LL_MAX_DRIVER_TORQUE_ENABLE"
  Switch86/1 -> Bus Creator4/6  "LL_MAX_LANE_WIDTH_ENABLE"
  Data Type Conversion89/1 -> Switch58/1, Switch58/2
  Switch56/1 -> Bus Creator4/14  "LL_LKAS_OUT_OF_CONTROL_TTLC"
  LLSMConClb2/1 -> Switch47/3
  Data Type Conversion25/1 -> Switch51/1, Switch51/2
  LL_RlsDet_tiTrqChkT_DISABLE=0.25/1 -> Switch38/3
  LL_TkOvStChk_tiTrqChkT_DEACTV=0.2/1 -> Switch16/3
  Data Type Conversion7/1 -> Switch40/2, Switch40/1
  Switch38/1 -> Bus Creator6/19  "LL_RlsDet_tiTrqChkT_DISABLE"
  Data Type Conversion5/1 -> Switch16/1, Switch16/2
  Switch16/1 -> Bus Creator6/17  "LL_TkOvStChk_tiTrqChkT_DEACTV"
  Switch40/1 -> Bus Creator6/18  "LL_TkOvStChk_tiTDelTime_DEACTV"
  Data Type Conversion9/1 -> Switch46/2, Switch46/1
  Data Type Conversion8/1 -> Switch44/2, Switch44/1
  Switch46/1 -> Bus Creator6/21  "LL_RlsDet_tiTDelTime_DISABLE"
  LL_RlsDet_tiTDelTime_DISABLE=20/1 -> Switch46/3
  LL_TkOvStChk_tiTDelTime_DEACTV=1/1 -> Switch40/3
  Data Type Conversion6/1 -> Switch38/1, Switch38/2
  Switch44/1 -> Bus Creator6/20  "LL_RlsDet_tiTrqChkT_EPS_DISABLE"
  LL_RlsDet_tiTrqChkT_EPS_DISABLE=0.5/1 -> Switch44/3
  LL_RlsDet_tiTDelTime_DISABLE=1/1 -> Switch1/3
  Switch1/1 -> Bus Creator6/22  "LL_HandsOff_TextTime"
  Data Type Conversion1/1 -> Switch1/1, Switch1/2
  Data Type Conversion2/1 -> Switch2/2, Switch2/1
  LL_RlsDet_tiTDelTime_DISABLE=2/1 -> Switch2/3
  Switch2/1 -> Bus Creator6/23  "LL_HandsOff_WarnTime"
  Switch3/1 -> Bus Creator6/24  "LL_HandsOff_ExitTime"
  LL_RlsDet_tiTDelTime_DISABLE=3/1 -> Switch3/3
  Data Type Conversion3/1 -> Switch3/1, Switch3/2
  Data Type Conversion4/1 -> Switch4/2, Switch4/1
  LL_RlsDet_tiTDelTime_DISABLE=4/1 -> Switch4/3
  Switch4/1 -> Bus Creator6/25  "LL_SingleLane_Disable_Swt"

== system LKAS_AutoSave_20220310_1755/LKAS/SignalBusCreator/DTC_Indicator ==
  Bus Creator11 : BusCreator  Inputs=2
  Constant{,2..21} (21 alike) : Constant  Value=0  OutDataTypeStr=uint8
  Mux : Mux  Inputs=16
  Mux1 : Mux  Inputs=5
  bsDTC_Indicator : Outport
  wires:
  Bus Creator11/1 -> bsDTC_Indicator/1  "bsDTC_Indicator"
  Mux/1 -> Bus Creator11/1  "LKAS_BSWDTC_Status"
  Constant/1 -> Mux/1  "CANEve_e_BusOff_PSA1CAN"
  Constant2/1 -> Mux/2  "CANEve_e_BusOff_SensorCAN"
  Constant4/1 -> Mux/4  "CANEve_e_Node_ESC_Validity"
  Constant3/1 -> Mux/3  "CANEve_e_Mute_PSA1CAN"
  Constant7/1 -> Mux/7  "CANEve_e_Node_TCU_Validity"
  Constant8/1 -> Mux/8  "CANEve_e_Node_GW_Validity"
  Constant6/1 -> Mux/6  "CANEve_e_Node_EMS_Validity"
  Constant5/1 -> Mux/5  "CANEve_e_Node_EPS_Validity"
  Constant13/1 -> Mux/13  "Reserved3"
  Constant14/1 -> Mux/14  "Reserved4"
  Constant16/1 -> Mux/16  "Reserved6"
  Constant15/1 -> Mux/15  "Reserved5"
  Constant11/1 -> Mux/11  "Reserved1"
  Constant12/1 -> Mux/12  "Reserved2"
  Constant10/1 -> Mux/10  "CANEve_e_Node_Camera_Validity"
  Constant9/1 -> Mux/9  "CANEve_e_Node_Radar_Validity"
  Constant17/1 -> Mux1/1  "ACC"
  Constant18/1 -> Mux1/2  "AEB"
  Constant19/1 -> Mux1/3  "LKA"
  Constant20/1 -> Mux1/4  "LDW"
  Constant21/1 -> Mux1/5  "TJA"
  Mux1/1 -> Bus Creator11/2  "Indicator_Status"

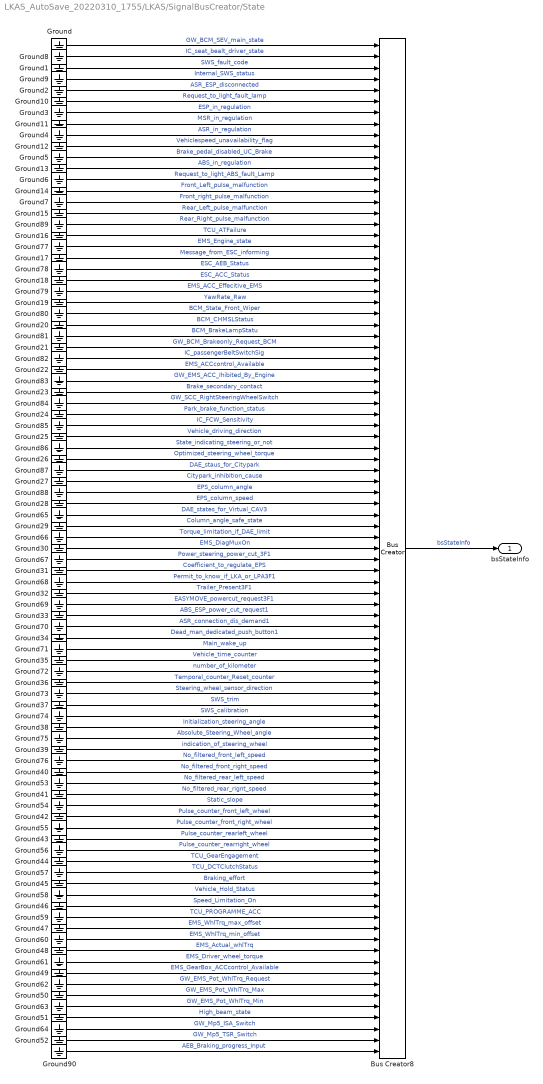
== system LKAS_AutoSave_20220310_1755/LKAS/SignalBusCreator/State ==
  Bus Creator8 : BusCreator  Inputs=91
  Ground{,1..90} (91 alike) : Ground
  bsStateInfo : Outport
  wires:
  Ground14/1 -> Bus Creator8/14  "Front_Left_pulse_malfunction"
  Ground8/1 -> Bus Creator8/2  "IC_seat_bealt_driver_state"
  Ground/1 -> Bus Creator8/1  "GW_BCM_SEV_main_state"
  Ground42/1 -> Bus Creator8/70  "Pulse_counter_front_left_wheel"
  Ground43/1 -> Bus Creator8/72  "Pulse_counter_rearleft_wheel"
  Ground12/1 -> Bus Creator8/10  "Vehiclespeed_unavailability_flag"
  Ground75/1 -> Bus Creator8/63  "Absolute_Steering_Wheel_angle"
  Ground71/1 -> Bus Creator8/55  "Main_wake_up"
  Ground44/1 -> Bus Creator8/74  "TCU_GearEngagement"
  Ground55/1 -> Bus Creator8/71  "Pulse_counter_front_right_wheel"
  Ground7/1 -> Bus Creator8/15  "Front_right_pulse_malfunction"
  Ground28/1 -> Bus Creator8/42  "EPS_column_speed"
  Ground79/1 -> Bus Creator8/23  "EMS_ACC_Effecitive_EMS"
  Ground77/1 -> Bus Creator8/19  "EMS_Engine_state"
  Ground80/1 -> Bus Creator8/25  "BCM_State_Front_Wiper"
  Ground41/1 -> Bus Creator8/68  "No_filtered_rear_rignt_speed"
  Ground67/1 -> Bus Creator8/47  "Power_steering_power_cut_3F1"
  Bus Creator8/1 -> bsStateInfo/1  "bsStateInfo"
  Ground90/1 -> Bus Creator8/91  "AEB_Braking_progress_Input"
  Ground38/1 -> Bus Creator8/62  "Initialization_steering_angle"
  Ground19/1 -> Bus Creator8/24  "YawRate_Raw"
  Ground83/1 -> Bus Creator8/31  "GW_EMS_ACC_Ihibited_By_Engine"
  Ground46/1 -> Bus Creator8/78  "Speed_Limitation_On"
  Ground51/1 -> Bus Creator8/88  "High_beam_state"
  Ground40/1 -> Bus Creator8/66  "No_filtered_front_right_speed"
  Ground3/1 -> Bus Creator8/7  "ESP_in_regulation"
  Ground36/1 -> Bus Creator8/58  "Temporal_counter_Reset_counter"
  Ground11/1 -> Bus Creator8/8  "MSR_in_regulation"
  Ground50/1 -> Bus Creator8/86  "GW_EMS_Pot_WhlTrq_Max"
  Ground10/1 -> Bus Creator8/6  "Request_to_light_fault_lamp"
  Ground13/1 -> Bus Creator8/12  "ABS_in_regulation"
  Ground5/1 -> Bus Creator8/11  "Brake_pedal_disabled_UC_Brake"
  Ground23/1 -> Bus Creator8/32  "Brake_secondary_contact"
  Ground60/1 -> Bus Creator8/81  "EMS_WhlTrq_min_offset"
  Ground15/1 -> Bus Creator8/16  "Rear_Left_pulse_malfunction"
  Ground24/1 -> Bus Creator8/34  "Park_brake_function_status"
  Ground6/1 -> Bus Creator8/13  "Request_to_light_ABS_fault_Lamp"
  Ground66/1 -> Bus Creator8/45  "Torque_limitation_if_DAE_limit"
  Ground72/1 -> Bus Creator8/57  "number_of_kilometer"
  Ground9/1 -> Bus Creator8/4  "Internal_SWS_status"
  Ground31/1 -> Bus Creator8/48  "Coefficient_to_regulate_EPS"
  Ground89/1 -> Bus Creator8/17  "Rear_Right_pulse_malfunction"
  Ground22/1 -> Bus Creator8/30  "EMS_ACCcontrol_Available"
  Ground73/1 -> Bus Creator8/59  "Steering_wheel_sensor_direction"
  Ground52/1 -> Bus Creator8/90  "GW_Mp5_TSR_Switch"
  Ground54/1 -> Bus Creator8/69  "Static_slope"
  Ground63/1 -> Bus Creator8/87  "GW_EMS_Pot_WhlTrq_Min"
  Ground25/1 -> Bus Creator8/36  "Vehicle_driving_direction"
  Ground69/1 -> Bus Creator8/51  "EASYMOVE_powercut_request3F1"
  Ground39/1 -> Bus Creator8/64  "indication_of_steering_wheel"
  Ground20/1 -> Bus Creator8/26  "BCM_CHMSLStatus"
  Ground57/1 -> Bus Creator8/75  "TCU_DCTClutchStatus"
  Ground27/1 -> Bus Creator8/40  "Citypark_inhibition_cause"
  Ground18/1 -> Bus Creator8/22  "ESC_ACC_Status"
  Ground65/1 -> Bus Creator8/43  "DAE_states_for_Virtual_CAV3"
  Ground84/1 -> Bus Creator8/33  "GW_SCC_RightSteeringWheelSwitch"
  Ground26/1 -> Bus Creator8/38  "Optimized_steering_wheel_torque"
  Ground33/1 -> Bus Creator8/52  "ABS_ESP_power_cut_request1"
  Ground17/1 -> Bus Creator8/20  "Message_from_ESC_informing"
  Ground29/1 -> Bus Creator8/44  "Column_angle_safe_state"
  Ground30/1 -> Bus Creator8/46  "EMS_DiagMuxOn"
  Ground68/1 -> Bus Creator8/49  "Permit_to_know_if_LKA_or_LPA3F1"
  Ground70/1 -> Bus Creator8/53  "ASR_connection_dis_demand1"
  Ground74/1 -> Bus Creator8/61  "SWS_calibration"
  Ground4/1 -> Bus Creator8/9  "ASR_in_regulation"
  Ground37/1 -> Bus Creator8/60  "SWS_trim"
  Ground53/1 -> Bus Creator8/67  "No_filtered_rear_left_speed"
  Ground2/1 -> Bus Creator8/5  "ASR_ESP_disconnected"
  Ground56/1 -> Bus Creator8/73  "Pulse_counter_rearright_wheel"
  Ground21/1 -> Bus Creator8/28  "GW_BCM_Brakeonly_Request_BCM"
  Ground59/1 -> Bus Creator8/79  "TCU_PROGRAMME_ACC"
  Ground47/1 -> Bus Creator8/80  "EMS_WhlTrq_max_offset"
  Ground45/1 -> Bus Creator8/76  "Braking_effort"
  Ground48/1 -> Bus Creator8/82  "EMS_Actual_whlTrq"
  Ground49/1 -> Bus Creator8/84  "EMS_GearBox_ACCcontrol_Available"
  Ground87/1 -> Bus Creator8/39  "DAE_staus_for_Citypark"
  Ground86/1 -> Bus Creator8/37  "State_indicating_steering_or_not"
  Ground85/1 -> Bus Creator8/35  "IC_FCW_Sensitivity"
  Ground78/1 -> Bus Creator8/21  "ESC_AEB_Status"
  Ground82/1 -> Bus Creator8/29  "IC_passengerBeltSwitchSig"
  Ground81/1 -> Bus Creator8/27  "BCM_BrakeLampStatu"
  Ground58/1 -> Bus Creator8/77  "Vehicle_Hold_Status"
  Ground64/1 -> Bus Creator8/89  "GW_Mp5_ISA_Switch"
  Ground35/1 -> Bus Creator8/56  "Vehicle_time_counter"
  Ground34/1 -> Bus Creator8/54  "Dead_man_dedicated_push_button1"
  Ground32/1 -> Bus Creator8/50  "Trailer_Present3F1"
  Ground61/1 -> Bus Creator8/83  "EMS_Driver_wheel_torque"
  Ground76/1 -> Bus Creator8/65  "No_filtered_front_left_speed"
  Ground62/1 -> Bus Creator8/85  "GW_EMS_Pot_WhlTrq_Request"
  Ground88/1 -> Bus Creator8/41  "EPS_column_angle"
  Ground16/1 -> Bus Creator8/18  "TCU_ATFailure"
  Ground1/1 -> Bus Creator8/3  "SWS_fault_code"

== system LKAS_AutoSave_20220310_1755/LKAS/LL/Human Machine Interface (HMI)/Subsystem ==
  LDW_STATE : Inport
  LKA_STATE : Inport  Port=2
  EPSInfo : Inport  Port=3
  SampleTime : Inport  Port=4
  HandsOff_Text : Inport  Port=5
  HandsOff_Warn : Inport  Port=6
  Abs : Abs
  Bus Selector2 : BusSelector  OutputSignals=EPS_LKA_State,EPS_SW_Trq
  Compare{1..2,4,7} (4 alike) : simulink/Logic and Bit Operations/Compare To Constant  relop===  const=3  OutDataTypeStr=boolean
  Compare3 : simulink/Logic and Bit Operations/Compare To Constant  relop===  const=1  OutDataTypeStr=boolean
  Compare5 : simulink/Logic and Bit Operations/Compare To Constant  relop===  const=4  OutDataTypeStr=boolean
  Compare6 : simulink/Logic and Bit Operations/Compare To Constant  relop===  const=5  OutDataTypeStr=boolean
  Compare8 : simulink/Logic and Bit Operations/Compare To Constant  relop===  const=4  OutDataTypeStr=boolean
  Compare9 : simulink/Logic and Bit Operations/Compare To Constant  relop===  const=5  OutDataTypeStr=boolean
  Constant : Constant  Value=0.25  OutDataTypeStr=single
  Constant1 : Constant  Value=0.5  OutDataTypeStr=single
  Logical Operator1 : Logic  Operator=OR  AllPortsSameDT=off  OutDataTypeStr=boolean
  Logical Operator2 : Logic  Inputs=3  AllPortsSameDT=off  OutDataTypeStr=boolean
  Logical Operator3 : Logic  Operator=OR  Inputs=6  AllPortsSameDT=off  OutDataTypeStr=boolean
  Relational Operator : RelationalOperator  Operator=<=  OutDataTypeStr=boolean  RndMeth=Nearest
  Sum Condition1 : Subsystem  TreatAsAtomicUnit=on
  Sum Condition2 : Subsystem  TreatAsAtomicUnit=on
  Switch : Switch  Criteria=u2 > Threshold
  HandsOff2_Warn : Outport
  HandsOff1_Text : Outport  Port=2
  wires:
  Sum Condition1/1(Out) -> HandsOff1_Text/1
  Bus Selector2/1 -> Compare3/1, Compare2/1, Compare1/1  "<EPS_LKA_State>"
  Constant/1 -> Switch/3
  EPSInfo/1 -> Bus Selector2/1
  Switch/1 -> Relational Operator/2
  Compare1/1 -> Switch/2
  Bus Selector2/2 -> Abs/1  "<EPS_SW_Trq>"
  Logical Operator2/1 -> Sum Condition1/Enable, Sum Condition2/Enable
  Logical Operator3/1 -> Logical Operator2/1
  Constant1/1 -> Switch/1
  Relational Operator/1 -> Logical Operator2/3
  Sum Condition2/1(Out) -> HandsOff2_Warn/1
  LDW_STATE/1 -> Compare4/1, Compare6/1, Compare5/1
  Compare4/1 -> Logical Operator3/3
  Compare5/1 -> Logical Operator3/2
  Compare6/1 -> Logical Operator3/1
  Abs/1 -> Relational Operator/1
  LKA_STATE/1 -> Compare9/1, Compare8/1, Compare7/1
  Compare9/1 -> Logical Operator3/4
  Compare8/1 -> Logical Operator3/5
  Compare7/1 -> Logical Operator3/6
  Compare2/1 -> Logical Operator1/1
  Compare3/1 -> Logical Operator1/2
  Logical Operator1/1 -> Logical Operator2/2
  SampleTime/1 -> Sum Condition2/1(SampleTime), Sum Condition1/1(SampleTime)
  HandsOff_Text/1 -> Sum Condition1/2(Sum)
  HandsOff_Warn/1 -> Sum Condition2/2(Sum)

== system LKAS_AutoSave_20220310_1755/LKAS/LL/LL Inputs Mapping/bsBCMInfo ==
  bsBCMInfoIn : Inport
  Bus Creator1 : BusCreator  Inputs=3
  Bus Selector1 : BusSelector  OutputSignals=BCM_Double_Light,BCM_Left_Light,BCM_Right_Light,BCM_LeftTurn_Switch,BCM_RightTurn_Switch
  Compare To Constant : simulink/Logic and Bit Operations/Compare To Constant  relop===  const=1  OutDataTypeStr=boolean
  Compare To Constant1 : simulink/Logic and Bit Operations/Compare To Constant  relop===  const=1  OutDataTypeStr=boolean
  Logical Operator : Logic  Operator=OR  AllPortsSameDT=off  OutDataTypeStr=boolean
  Logical Operator1 : Logic  Operator=OR  AllPortsSameDT=off  OutDataTypeStr=boolean
  bsBCMInfoOut : Outport
  wires:
  Bus Selector1/3 -> Logical Operator1/1  "<BCM_Right_Light>"
  Bus Selector1/2 -> Logical Operator/1  "<BCM_Left_Light>"
  Bus Creator1/1 -> bsBCMInfoOut/1
  Bus Selector1/1 -> Bus Creator1/1  "<BCM_Double_Light>"
  bsBCMInfoIn/1 -> Bus Selector1/1
  Bus Selector1/4 -> Compare To Constant/1  "<BCM_LeftTurn_Switch>"
  Bus Selector1/5 -> Compare To Constant1/1  "<BCM_RightTurn_Switch>"
  Compare To Constant/1 -> Logical Operator/2
  Compare To Constant1/1 -> Logical Operator1/2
  Logical Operator/1 -> Bus Creator1/2  "BCM_Left_Light"
  Logical Operator1/1 -> Bus Creator1/3  "BCM_Right_Light"

== system LKAS_AutoSave_20220310_1755/LKAS/LL/LL Inputs Mapping/bsEPSInfo ==
  bsEPSInfoIn : Inport
  Bus Creator4 : BusCreator  Inputs=11
  Bus Selector1 : BusSelector  OutputSignals=EPS_LKA_State,EPS_SW_Trq,EPS_Trq_State,SAS_Clb_State,SAS_Trim_State,SWS_Failure_Status,EPS_TrqLim_State,EPS_LKA_Current,EPS_SWHold_State,EPS_Driver_Override,EPS_ESA_State
  bsEPSInfoOut : Outport
  wires:
  Bus Selector1/9 -> Bus Creator4/9  "<EPS_SWHold_State>"
  Bus Selector1/8 -> Bus Creator4/8  "<EPS_LKA_Current>"
  Bus Selector1/7 -> Bus Creator4/7  "<EPS_TrqLim_State>"
  Bus Selector1/5 -> Bus Creator4/5  "<SAS_Trim_State>"
  Bus Selector1/4 -> Bus Creator4/4  "<SAS_Clb_State>"
  Bus Selector1/3 -> Bus Creator4/3  "<EPS_Trq_State>"
  Bus Creator4/1 -> bsEPSInfoOut/1
  Bus Selector1/1 -> Bus Creator4/1  "<EPS_LKA_State>"
  Bus Selector1/2 -> Bus Creator4/2  "<EPS_SW_Trq>"
  bsEPSInfoIn/1 -> Bus Selector1/1
  Bus Selector1/6 -> Bus Creator4/6  "<SWS_Failure_Status>"
  Bus Selector1/10 -> Bus Creator4/10  "<EPS_Driver_Override>"
  Bus Selector1/11 -> Bus Creator4/11  "<EPS_ESA_State>"

== system LKAS_AutoSave_20220310_1755/LKAS/LL/LL Inputs Mapping/bsLaneInfo ==
  bsLLClb : Inport
  bsLaneInfoIn : Inport  Port=2
  Bus Creator : BusCreator  Inputs=5
  Bus Selector1 : BusSelector  OutputSignals=bsFusL0Info,bsFusR0Info,bsFusL1Info,bsFusR1Info,Fusion_AdditionalInf
  LaneSelect : Subsystem
  "LanesReconstruct " : Subsystem
  bsLaneInfoOut : Outport
  wires:
  Bus Creator/1 -> bsLaneInfoOut/1
  Bus Selector1/4 -> LaneSelect/4(bsFusR1Info)  "<bsFusR1Info>"
  Bus Selector1/3 -> LaneSelect/3(bsFusL1Info)  "<bsFusL1Info>"
  Bus Selector1/2 -> LaneSelect/2(bsFusR0Info)  "<bsFusR0Info>"
  Bus Selector1/1 -> LaneSelect/1(bsFusL0Info)  "<bsFusL0Info>"
  LaneSelect/4(bsR1Info) -> "LanesReconstruct "/5(bsR1Info)
  LaneSelect/3(bsL1Info) -> "LanesReconstruct "/4(bsL1Info)
  LaneSelect/2(bsR0Info) -> "LanesReconstruct "/3(bsR0Info)
  LaneSelect/1(bsL0Info) -> "LanesReconstruct "/2(bsL0Info)
  "LanesReconstruct "/4(bsR1InfoR) -> Bus Creator/4  "bsR1Info"
  "LanesReconstruct "/3(bsL1InfoR) -> Bus Creator/3  "bsL1Info"
  "LanesReconstruct "/2(bsR0InfoR) -> Bus Creator/2  "bsR0Info"
  "LanesReconstruct "/1(bsL0InfoR) -> Bus Creator/1  "bsL0Info"
  Bus Selector1/5 -> Bus Creator/5  "<Fusion_AdditionalInf>"
  bsLaneInfoIn/1 -> Bus Selector1/1
  bsLLClb/1 -> "LanesReconstruct "/1(bsLLClb)

== system LKAS_AutoSave_20220310_1755/LKAS/LL/LL Inputs Mapping/bsMP5Info ==
  note: LkaFcnConf
      | 0: OFF
      | 1: LDW-声音
      | 2: LDW-振动
      | 3: LDW-声音+振动
      | 4: LKA-声音
      | 5: LKA-振动
      | 6: LKA-声音+振动
      | 7: LDW-声音-ICA
      | 8: LDW-振动-ICA
      | 9: LDW-声音+振动-ICA
      | 10: LKA-声音-ICA
      | 11: LKA-振动-ICA
      | 12: LKA-声音+振动-ICA
  bsMP5InfoIn : Inport
  Add : Sum
  Add1 : Sum  Inputs=+-  OutMin=0  OutMax=12
  Bus Creator : BusCreator  Inputs=5
  Bus Selector1 : BusSelector  OutputSignals=LkaFcnConf,LKA_Main_Switch,LKA_Mode,LDW_Warn_Mode,APA_AutoPark_WorkSt,MP5_Work_State
  Constant1 : Constant  OutDataTypeStr=uint8
  Constant2 : Constant  Value=6  OutDataTypeStr=uint8
  Constant3 : Constant  OutDataTypeStr=uint8
  Constant4 : Constant  Value=0  OutDataTypeStr=uint8
  Constant5 : Constant  Value=3  OutDataTypeStr=uint8
  Constant6 : Constant  OutDataTypeStr=uint8
  Constant7 : Constant  Value=3  OutDataTypeStr=uint8
  Divide : Product  Inputs=**  OutDataTypeStr=uint8
  Divide1 : Product  Inputs=*/
  Logical Operator : Logic  Operator=OR  AllPortsSameDT=off  OutDataTypeStr=boolean
  Max : MinMax  Function=max  Inputs=2
  Max1 : MinMax  Function=max  Inputs=2
  Mod : Math  Operator=mod  SaturateOnIntegerOverflow=on
  Mod1 : Math  Operator=mod  SaturateOnIntegerOverflow=on
  Saturation : Saturate  UpperLimit=12  LowerLimit=0
  Saturation1 : Saturate  UpperLimit=12  LowerLimit=1
  Switch : Switch  Criteria=u2 > Threshold
  bsMP5InfoOut : Outport
  wires:
  bsMP5InfoIn/1 -> Bus Selector1/1
  Divide/1 -> Bus Creator/2  "LKA_Mode"
  Bus Selector1/2 -> Logical Operator/2  "<LKA_Main_Switch>"
  Add/1 -> Divide/2
  Bus Selector1/3 -> Max/2  "<LKA_Mode>"
  Constant6/1 -> Add/2
  Bus Selector1/1 -> Switch/2, Saturation1/1  "<LkaFcnConf>"
  Constant1/1 -> Add1/2
  Add1/1 -> Saturation/1
  Constant2/1 -> Mod/2
  Constant3/1 -> Switch/1
  Constant4/1 -> Switch/3
  Switch/1 -> Logical Operator/1
  Logical Operator/1 -> Divide/1, Bus Creator/1  "LKA_Main_Switch"
  Bus Selector1/5 -> Bus Creator/4  "<APA_AutoPark_WorkSt>"
  Bus Selector1/6 -> Bus Creator/5  "<MP5_Work_State>"
  Bus Creator/1 -> bsMP5InfoOut/1
  Saturation/1 -> Mod1/1, Mod/1
  Mod/1 -> Divide1/1
  Constant5/1 -> Divide1/2
  Divide1/1 -> Max/1
  Max/1 -> Add/1
  Constant7/1 -> Mod1/2
  Mod1/1 -> Max1/1
  Bus Selector1/4 -> Max1/2  "<LDW_Warn_Mode>"
  Max1/1 -> Bus Creator/3  "LDW_Warn_Mode"
  Saturation1/1 -> Add1/1

== system LKAS_AutoSave_20220310_1755/LKAS/LL/LL Inputs Mapping/bsPTState ==
  bsPTStateIn : Inport
  Bus Creator3 : BusCreator  Inputs=3
  Bus Selector1 : BusSelector  OutputSignals=AccPedal_Pos,TCU_ActualGear,TCU_Available
  Constant1 : Constant  Value=0  OutDataTypeStr=uint8
  Constant3 : Constant  Value=3  OutDataTypeStr=uint8
  Multiport Switch : MultiPortSwitch  DataPortOrder=Zero-based contiguous  Inputs=11  zeroidx=on
  bsPTStateOut : Outport
  wires:
  Bus Creator3/1 -> bsPTStateOut/1
  Bus Selector1/1 -> Bus Creator3/1  "<AccPedal_Pos>"
  bsPTStateIn/1 -> Bus Selector1/1
  Multiport Switch/1 -> Bus Creator3/2  "TCU_ActualGear"
  Constant3/1 -> Multiport Switch/11, Multiport Switch/10, Multiport Switch/9, Multiport Switch/6, Multiport Switch/5, Multiport Switch/4, Multiport Switch/3
  Bus Selector1/2 -> Multiport Switch/1  "<TCU_ActualGear>"
  Constant1/1 -> Multiport Switch/12, Multiport Switch/8, Multiport Switch/7, Multiport Switch/2
  Bus Selector1/3 -> Bus Creator3/3  "<TCU_Available>"

== system LKAS_AutoSave_20220310_1755/LKAS/LL/LL Inputs Mapping/bsSWAInfo ==
  bsSWAInfoIn : Inport
  Bus Creator : BusCreator  Inputs=4
  Bus Selector1 : BusSelector  OutputSignals=EPS_SteeringAngle_Flag,EPS_SteeringAngle,SW_Angle,SW_Angle_Speed
  bsSWAInfoOut : Outport
  wires:
  Bus Creator/1 -> bsSWAInfoOut/1
  Bus Selector1/4 -> Bus Creator/4  "<SW_Angle_Speed>"
  Bus Selector1/3 -> Bus Creator/3  "<SW_Angle>"
  bsSWAInfoIn/1 -> Bus Selector1/1
  Bus Selector1/2 -> Bus Creator/2  "<EPS_SteeringAngle>"
  Bus Selector1/1 -> Bus Creator/1  "<EPS_SteeringAngle_Flag>"
